simulink model "Ef_b"  (R2017a)
settings: Solver=VariableStepAuto  StartTime=0.0  StopTime=50  RelTol=1e-3
InitFcn:
  | m1 = .35;
  | m2 = 2;
  | l = .5;
  | g = 9.8;
  | ze = l/2;
  | 
  | C1 = 3/(m2*l^2+3*m1*ze^2);
  | 
  | tr_th = 1;
  | h_th = .707;
  | Wn_th = 2.2 / tr_th;
  | kd_th = 2*h_th*Wn_th/C1/l;
  | kp_th = Wn_th^2/(C1*l);
  | 
  | tr_z = 5*tr_th;
  | h = .707;
  | Wn = 2.2 / tr_z;
  | 
  | K = -Wn^2/9.81;
  | a = -K / ((1*h*Wn*1.5+.1)/(1.5*9.81));
  | K = -.0197;
  | a = .3;
  | 
  | E_param
settings Model: Creator=Mat Haskell  LastModifiedBy=Mat Haskell

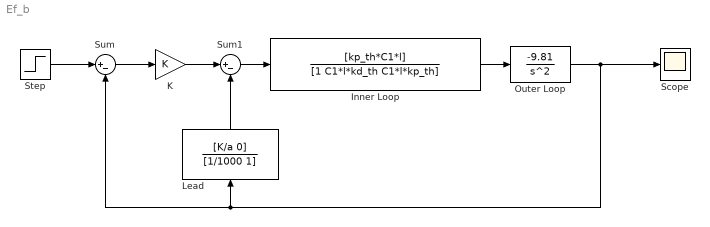
== system Ef_b ==
  Inner Loop : TransferFcn  Numerator=[kp_th*C1*l]  Denominator=[1 C1*l*kd_th C1*l*kp_th]
  K : Gain  Gain=K
  Lead : TransferFcn  Numerator=[K/a 0]  Denominator=[1/1000 1]
  Outer Loop : TransferFcn  Numerator=[-9.81]  Denominator=[1 0 0]
  Scope : Scope
  Step : Step  After=.25  SampleTime=0
  Sum : Sum  Inputs=|+-
  Sum1 : Sum  Inputs=|+-
  wires:
  Lead/1 -> Sum1/2
  Step/1 -> Sum/1
  Sum1/1 -> Inner Loop/1
  Inner Loop/1 -> Outer Loop/1
  Outer Loop/1 -> Sum/2, Lead/1, Scope/1
  K/1 -> Sum1/1
  Sum/1 -> K/1
